simulink model "Memory_Blocks"  (Simulink 8.1)
settings: Solver=ode45  StartTime=0.0  StopTime=10.0  RelTol=1e-3
libraries: Common_Library x36, simulink_extras x9, commutil2 x2
settings Model: Creator=uzivatel  LastModifiedBy=uzivatel
settings DataIOCC: SignalLoggingSaveFormat=Dataset
settings OptimizationCC: ExpressionDepthLimit=128
settings DebuggingCC: FcnCallInpInsideContextMsg=EnableAllAsError
settings GRTTargetCC: CombineOutputUpdateFcns=on  GRTInterface=off

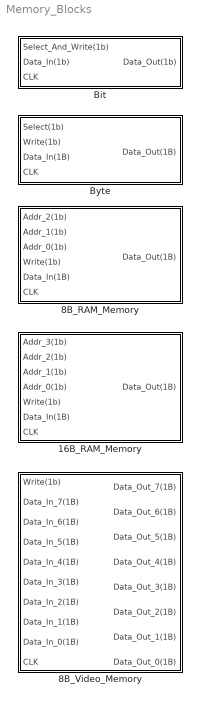
== system Memory_Blocks ==
  16B_RAM_Memory : Subsystem
  8B_RAM_Memory : Subsystem
  8B_Video_Memory : Subsystem
  Bit : Subsystem
  Byte : Subsystem

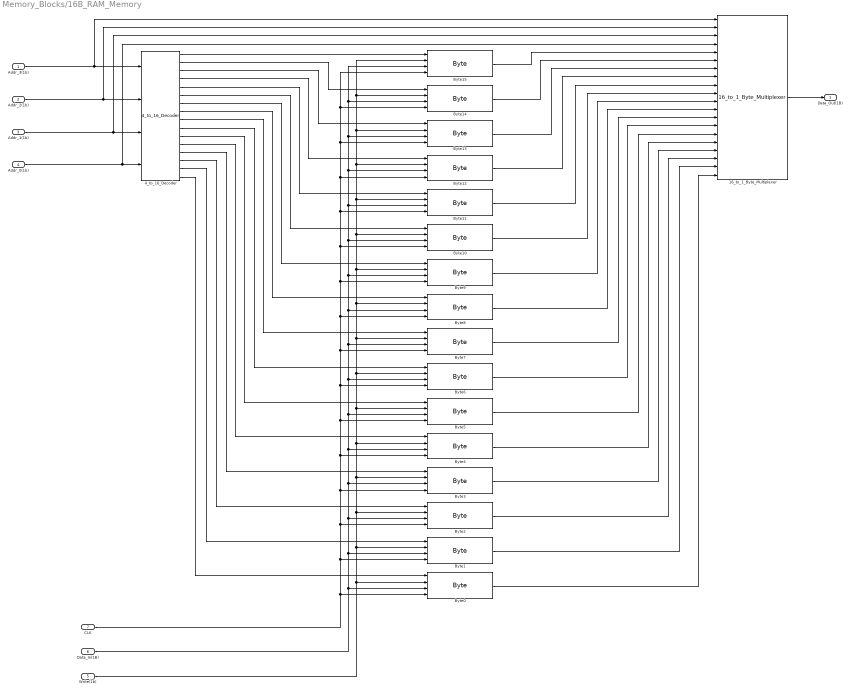
== system Memory_Blocks/16B_RAM_Memory ==
  Addr_3(1b) : Inport
  Addr_2(1b) : Inport  Port=2
  Addr_1(1b) : Inport  Port=3
  Addr_0(1b) : Inport  Port=4
  Write(1b) : Inport  Port=5
  Data_In(1B) : Inport  Port=6
  CLK : Inport  Port=7  OutDataTypeStr=double
  16_to_1_Byte_Multiplexer : Common_Library/Multiplexers/16_to_1_Byte_Multiplexer
  4_to_16_Decoder : Common_Library/Decoders/4_to_16_Decoder
  Byte{0..15} (16 alike) : Common_Library/Memory_Blocks/Byte
  Data_Out(1B) : Outport
  wires:
  16_to_1_Byte_Multiplexer/1 -> Data_Out(1B)/1
  Byte0/1 -> 16_to_1_Byte_Multiplexer/20
  Byte1/1 -> 16_to_1_Byte_Multiplexer/19
  Byte2/1 -> 16_to_1_Byte_Multiplexer/18
  Byte3/1 -> 16_to_1_Byte_Multiplexer/17
  Byte4/1 -> 16_to_1_Byte_Multiplexer/16
  Byte5/1 -> 16_to_1_Byte_Multiplexer/15
  Byte6/1 -> 16_to_1_Byte_Multiplexer/14
  Byte7/1 -> 16_to_1_Byte_Multiplexer/13
  Byte8/1 -> 16_to_1_Byte_Multiplexer/12
  Byte9/1 -> 16_to_1_Byte_Multiplexer/11
  Byte10/1 -> 16_to_1_Byte_Multiplexer/10
  Byte11/1 -> 16_to_1_Byte_Multiplexer/9
  Byte12/1 -> 16_to_1_Byte_Multiplexer/8
  Byte13/1 -> 16_to_1_Byte_Multiplexer/7
  Byte14/1 -> 16_to_1_Byte_Multiplexer/6
  Byte15/1 -> 16_to_1_Byte_Multiplexer/5
  4_to_16_Decoder/16 -> Byte0/1
  4_to_16_Decoder/15 -> Byte1/1
  4_to_16_Decoder/14 -> Byte2/1
  4_to_16_Decoder/13 -> Byte3/1
  4_to_16_Decoder/12 -> Byte4/1
  4_to_16_Decoder/11 -> Byte5/1
  4_to_16_Decoder/10 -> Byte6/1
  4_to_16_Decoder/9 -> Byte7/1
  4_to_16_Decoder/8 -> Byte8/1
  4_to_16_Decoder/7 -> Byte9/1
  4_to_16_Decoder/6 -> Byte10/1
  4_to_16_Decoder/5 -> Byte11/1
  4_to_16_Decoder/4 -> Byte12/1
  4_to_16_Decoder/3 -> Byte13/1
  4_to_16_Decoder/2 -> Byte14/1
  Addr_3(1b)/1 -> 16_to_1_Byte_Multiplexer/1, 4_to_16_Decoder/1
  4_to_16_Decoder/1 -> Byte15/1
  Write(1b)/1 -> Byte15/2, Byte14/2, Byte13/2, Byte12/2, Byte11/2, Byte10/2, Byte9/2, Byte8/2, Byte7/2, Byte6/2, Byte5/2, Byte4/2, Byte3/2, Byte2/2, Byte1/2, Byte0/2
  Data_In(1B)/1 -> Byte15/3, Byte14/3, Byte13/3, Byte12/3, Byte11/3, Byte10/3, Byte9/3, Byte8/3, Byte7/3, Byte6/3, Byte5/3, Byte4/3, Byte3/3, Byte2/3, Byte1/3, Byte0/3
  CLK/1 -> Byte15/4, Byte14/4, Byte13/4, Byte12/4, Byte11/4, Byte10/4, Byte9/4, Byte8/4, Byte7/4, Byte6/4, Byte5/4, Byte4/4, Byte3/4, Byte2/4, Byte1/4, Byte0/4
  Addr_2(1b)/1 -> 16_to_1_Byte_Multiplexer/2, 4_to_16_Decoder/2
  Addr_1(1b)/1 -> 16_to_1_Byte_Multiplexer/3, 4_to_16_Decoder/3
  Addr_0(1b)/1 -> 16_to_1_Byte_Multiplexer/4, 4_to_16_Decoder/4

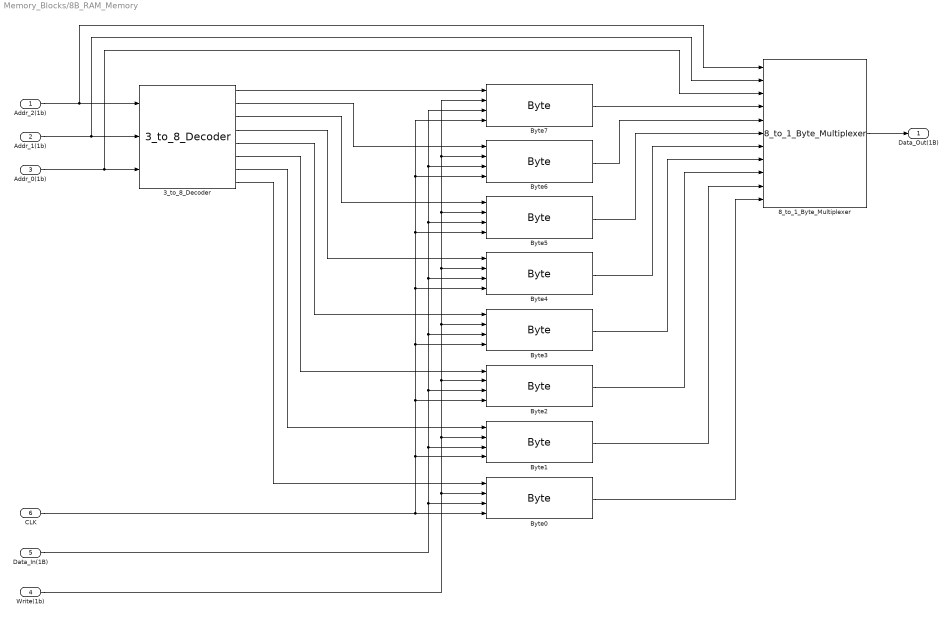
== system Memory_Blocks/8B_RAM_Memory ==
  Addr_2(1b) : Inport
  Addr_1(1b) : Inport  Port=2
  Addr_0(1b) : Inport  Port=3
  Write(1b) : Inport  Port=4
  Data_In(1B) : Inport  Port=5
  CLK : Inport  Port=6  OutDataTypeStr=double
  3_to_8_Decoder : Common_Library/Decoders/3_to_8_Decoder
  8_to_1_Byte_Multiplexer : Common_Library/Multiplexers/8_to_1_Byte_Multiplexer
  Byte{0..7} (8 alike) : Common_Library/Memory_Blocks/Byte
  Data_Out(1B) : Outport
  wires:
  8_to_1_Byte_Multiplexer/1 -> Data_Out(1B)/1
  Byte0/1 -> 8_to_1_Byte_Multiplexer/11
  Byte1/1 -> 8_to_1_Byte_Multiplexer/10
  Byte2/1 -> 8_to_1_Byte_Multiplexer/9
  Byte3/1 -> 8_to_1_Byte_Multiplexer/8
  Byte4/1 -> 8_to_1_Byte_Multiplexer/7
  Byte5/1 -> 8_to_1_Byte_Multiplexer/6
  Byte6/1 -> 8_to_1_Byte_Multiplexer/5
  Byte7/1 -> 8_to_1_Byte_Multiplexer/4
  3_to_8_Decoder/8 -> Byte0/1
  3_to_8_Decoder/7 -> Byte1/1
  3_to_8_Decoder/6 -> Byte2/1
  3_to_8_Decoder/5 -> Byte3/1
  3_to_8_Decoder/4 -> Byte4/1
  3_to_8_Decoder/3 -> Byte5/1
  3_to_8_Decoder/2 -> Byte6/1
  3_to_8_Decoder/1 -> Byte7/1
  Write(1b)/1 -> Byte7/2, Byte6/2, Byte5/2, Byte4/2, Byte3/2, Byte2/2, Byte1/2, Byte0/2
  Data_In(1B)/1 -> Byte7/3, Byte6/3, Byte5/3, Byte4/3, Byte3/3, Byte2/3, Byte1/3, Byte0/3
  CLK/1 -> Byte7/4, Byte6/4, Byte5/4, Byte4/4, Byte3/4, Byte2/4, Byte1/4, Byte0/4
  Addr_2(1b)/1 -> 8_to_1_Byte_Multiplexer/1, 3_to_8_Decoder/1
  Addr_1(1b)/1 -> 8_to_1_Byte_Multiplexer/2, 3_to_8_Decoder/2
  Addr_0(1b)/1 -> 8_to_1_Byte_Multiplexer/3, 3_to_8_Decoder/3

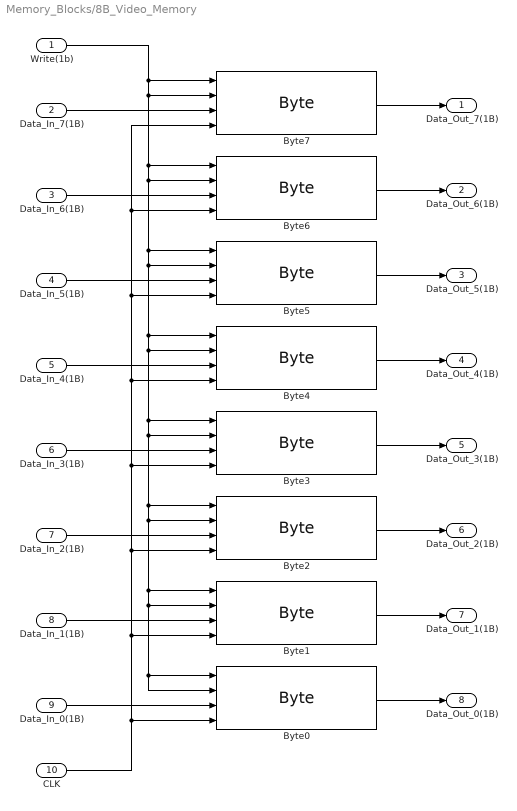
== system Memory_Blocks/8B_Video_Memory ==
  Write(1b) : Inport
  Data_In_7(1B) : Inport  Port=2
  Data_In_6(1B) : Inport  Port=3
  Data_In_5(1B) : Inport  Port=4
  Data_In_4(1B) : Inport  Port=5
  Data_In_3(1B) : Inport  Port=6
  Data_In_2(1B) : Inport  Port=7
  Data_In_1(1B) : Inport  Port=8
  Data_In_0(1B) : Inport  Port=9
  CLK : Inport  Port=10  OutDataTypeStr=double
  Byte{0..7} (8 alike) : Common_Library/Memory_Blocks/Byte
  Data_Out_7(1B) : Outport
  Data_Out_6(1B) : Outport  Port=2
  Data_Out_5(1B) : Outport  Port=3
  Data_Out_4(1B) : Outport  Port=4
  Data_Out_3(1B) : Outport  Port=5
  Data_Out_2(1B) : Outport  Port=6
  Data_Out_1(1B) : Outport  Port=7
  Data_Out_0(1B) : Outport  Port=8
  wires:
  Byte1/1 -> Data_Out_1(1B)/1
  Byte2/1 -> Data_Out_2(1B)/1
  Byte3/1 -> Data_Out_3(1B)/1
  Byte4/1 -> Data_Out_4(1B)/1
  Byte5/1 -> Data_Out_5(1B)/1
  Byte6/1 -> Data_Out_6(1B)/1
  Byte7/1 -> Data_Out_7(1B)/1
  Write(1b)/1 -> Byte0/2, Byte0/1, Byte1/2, Byte1/1, Byte2/2, Byte2/1, Byte3/2, Byte3/1, Byte4/2, Byte4/1, Byte5/2, Byte5/1, Byte6/2, Byte6/1, Byte7/2, Byte7/1
  CLK/1 -> Byte7/4, Byte6/4, Byte5/4, Byte4/4, Byte3/4, Byte2/4, Byte1/4, Byte0/4
  Byte0/1 -> Data_Out_0(1B)/1
  Data_In_7(1B)/1 -> Byte7/3
  Data_In_6(1B)/1 -> Byte6/3
  Data_In_5(1B)/1 -> Byte5/3
  Data_In_4(1B)/1 -> Byte4/3
  Data_In_3(1B)/1 -> Byte3/3
  Data_In_2(1B)/1 -> Byte2/3
  Data_In_1(1B)/1 -> Byte1/3
  Data_In_0(1B)/1 -> Byte0/3

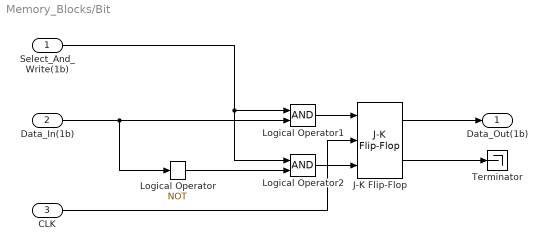
== system Memory_Blocks/Bit ==
  Select_And_Write(1b) : Inport  OutDataTypeStr=boolean
  Data_In(1b) : Inport  Port=2  OutDataTypeStr=boolean
  CLK : Inport  Port=3  OutDataTypeStr=double
  J-K Flip-Flop : simulink_extras/Flip Flops/J-K Flip-Flop  initial_condition=0
  Logical Operator : Logic  Operator=NOT  IconShape=distinctive  AllPortsSameDT=off  OutDataTypeStr=boolean
  Logical Operator1 : Logic  IconShape=distinctive  AllPortsSameDT=off  OutDataTypeStr=boolean
  Logical Operator2 : Logic  IconShape=distinctive  AllPortsSameDT=off  OutDataTypeStr=boolean
  Terminator : Terminator
  Data_Out(1b) : Outport
  wires:
  Data_In(1b)/1 -> Logical Operator/1, Logical Operator1/2
  J-K Flip-Flop/2 -> Terminator/1
  J-K Flip-Flop/1 -> Data_Out(1b)/1
  CLK/1 -> J-K Flip-Flop/2
  Select_And_Write(1b)/1 -> Logical Operator2/1, Logical Operator1/1
  Logical Operator/1 -> Logical Operator2/2
  Logical Operator1/1 -> J-K Flip-Flop/1
  Logical Operator2/1 -> J-K Flip-Flop/3

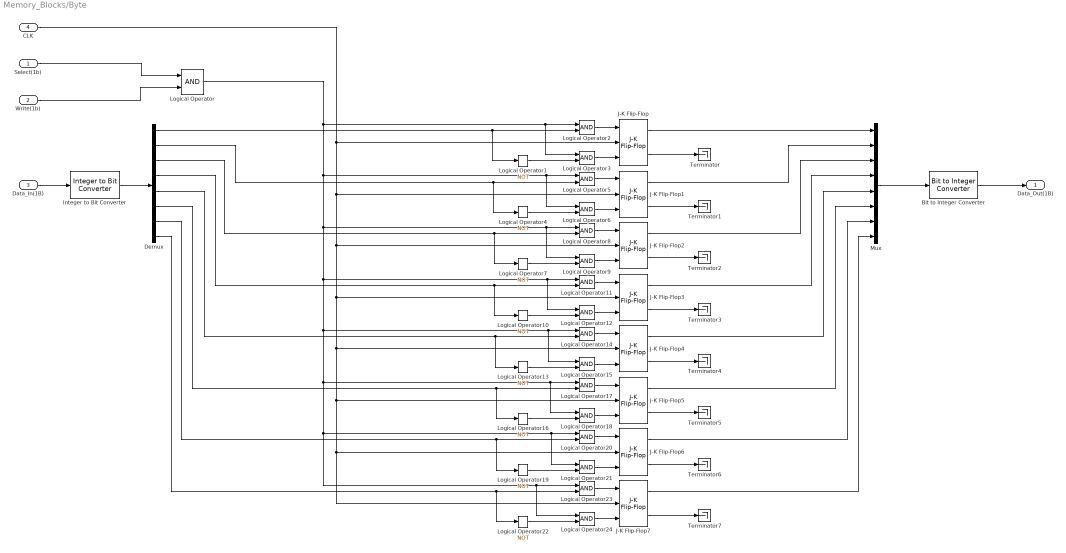
== system Memory_Blocks/Byte ==
  Select(1b) : Inport
  Write(1b) : Inport  Port=2
  Data_In(1B) : Inport  Port=3
  CLK : Inport  Port=4  OutDataTypeStr=double
  Bit to Integer Converter : commutil2/Bit to Integer Converter  nbits=8  bitOrder=MSB first  signedOutputValues=Unsigned  outDtype=uint8  outDtypeSigned=Inherit via internal rule
  Demux : Demux  Outputs=8
  Integer to Bit Converter : commutil2/Integer to Bit Converter  nbits=8  signedInputValues=Unsigned  bitOrder=MSB first  outDtype=boolean
  J-K Flip-Flop{,1..7} (8 alike) : simulink_extras/Flip Flops/J-K Flip-Flop  initial_condition=0
  Logical Operator{,2..3,5..6,8..9,11..12,14..15,17..18,20..21,23..24} (17 alike) : Logic  IconShape=distinctive  AllPortsSameDT=off  OutDataTypeStr=boolean
  Logical Operator{1,4,7,10,13,16,19,22} (8 alike) : Logic  Operator=NOT  IconShape=distinctive  AllPortsSameDT=off  OutDataTypeStr=boolean
  Mux : Mux  Inputs=8
  Terminator{,1..7} (8 alike) : Terminator
  Data_Out(1B) : Outport
  wires:
  Write(1b)/1 -> Logical Operator/2
  Select(1b)/1 -> Logical Operator/1
  Data_In(1B)/1 -> Integer to Bit Converter/1
  Mux/1 -> Bit to Integer Converter/1
  J-K Flip-Flop7/1 -> Mux/8
  J-K Flip-Flop6/1 -> Mux/7
  J-K Flip-Flop5/1 -> Mux/6
  J-K Flip-Flop4/1 -> Mux/5
  J-K Flip-Flop3/1 -> Mux/4
  J-K Flip-Flop2/1 -> Mux/3
  J-K Flip-Flop1/1 -> Mux/2
  J-K Flip-Flop/1 -> Mux/1
  Integer to Bit Converter/1 -> Demux/1
  Bit to Integer Converter/1 -> Data_Out(1B)/1
  Demux/1 -> Logical Operator1/1, Logical Operator2/2
  J-K Flip-Flop/2 -> Terminator/1
  Logical Operator1/1 -> Logical Operator3/2
  Logical Operator2/1 -> J-K Flip-Flop/1
  Logical Operator3/1 -> J-K Flip-Flop/3
  Demux/2 -> Logical Operator4/1, Logical Operator5/2
  J-K Flip-Flop1/2 -> Terminator1/1
  Logical Operator4/1 -> Logical Operator6/2
  Logical Operator5/1 -> J-K Flip-Flop1/1
  Logical Operator6/1 -> J-K Flip-Flop1/3
  Demux/3 -> Logical Operator7/1, Logical Operator8/2
  J-K Flip-Flop2/2 -> Terminator2/1
  Logical Operator7/1 -> Logical Operator9/2
  Logical Operator8/1 -> J-K Flip-Flop2/1
  Logical Operator9/1 -> J-K Flip-Flop2/3
  Demux/4 -> Logical Operator11/2, Logical Operator10/1
  J-K Flip-Flop3/2 -> Terminator3/1
  Logical Operator10/1 -> Logical Operator12/2
  Logical Operator11/1 -> J-K Flip-Flop3/1
  Logical Operator12/1 -> J-K Flip-Flop3/3
  Demux/5 -> Logical Operator14/2, Logical Operator13/1
  J-K Flip-Flop4/2 -> Terminator4/1
  Logical Operator13/1 -> Logical Operator15/2
  Logical Operator14/1 -> J-K Flip-Flop4/1
  Logical Operator15/1 -> J-K Flip-Flop4/3
  Demux/6 -> Logical Operator17/2, Logical Operator16/1
  J-K Flip-Flop5/2 -> Terminator5/1
  Logical Operator16/1 -> Logical Operator18/2
  Logical Operator17/1 -> J-K Flip-Flop5/1
  Logical Operator18/1 -> J-K Flip-Flop5/3
  Demux/7 -> Logical Operator19/1, Logical Operator20/2
  J-K Flip-Flop6/2 -> Terminator6/1
  Logical Operator19/1 -> Logical Operator21/2
  Logical Operator20/1 -> J-K Flip-Flop6/1
  Logical Operator21/1 -> J-K Flip-Flop6/3
  Demux/8 -> Logical Operator22/1, Logical Operator23/2
  J-K Flip-Flop7/2 -> Terminator7/1
  CLK/1 -> J-K Flip-Flop6/2, J-K Flip-Flop7/2, J-K Flip-Flop5/2, J-K Flip-Flop4/2, J-K Flip-Flop3/2, J-K Flip-Flop2/2, J-K Flip-Flop1/2, J-K Flip-Flop/2
  Logical Operator/1 -> Logical Operator24/1, Logical Operator23/1, Logical Operator21/1, Logical Operator20/1, Logical Operator17/1, Logical Operator18/1, Logical Operator15/1, Logical Operator14/1, Logical Operator12/1, Logical Operator11/1, Logical Operator9/1, Logical Operator8/1, Logical Operator6/1, Logical Operator5/1, Logical Operator3/1, Logical Operator2/1
  Logical Operator22/1 -> Logical Operator24/2
  Logical Operator23/1 -> J-K Flip-Flop7/1
  Logical Operator24/1 -> J-K Flip-Flop7/3
